simulink model "validacao_dados_degrau"  (R2021a)
settings: Solver=ode45  StartTime=0.0  StopTime=0.7  RelTol=1e-3
values from neighbouring files (symbols this model uses):
  tau_area = A0 / y_inf    [labeca_02_validacao_26_09.m]
  tau_nep = 1/a    [labeca_02_validacao_26_09.m]
undefined symbols (not defined in the file or in its folder): K_degrau
settings Model: Creator=Guilherme  LastModifiedBy=Guilherme
settings DebuggingCC: UnconnectedInputMsg=none  UnconnectedOutputMsg=none  UnconnectedLineMsg=none
settings ModelReferenceCC: EnableRefExpFcnMdlSchedulingChecks=off
settings RTWCC: Description=Generic Real-Time Target  GPUComputeCapability=5.0  DLArmComputeVersion=20.02.1

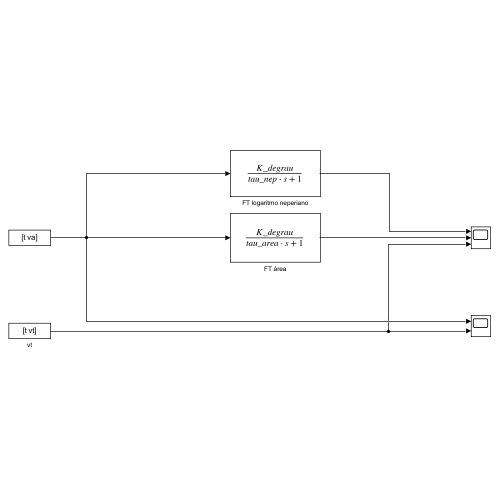
[thumbnail: Simulink's stored preview of the top-level diagram]
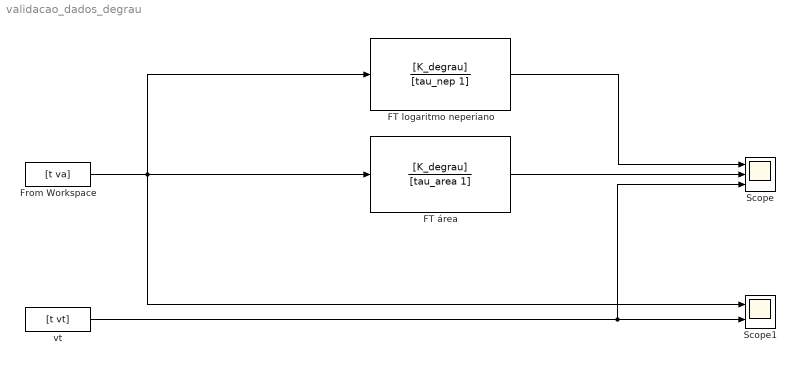
== system validacao_dados_degrau ==
  FT logaritmo neperiano : TransferFcn  Numerator=[K_degrau]  Denominator=[tau_nep 1]
  FT área : TransferFcn  Numerator=[K_degrau]  Denominator=[tau_area 1]
  From Workspace : FromWorkspace  VariableName=[t va]
  Scope : Scope  NumInputPorts=3
  Scope1 : Scope  NumInputPorts=2
  vt : FromWorkspace  VariableName=[t vt]
  wires:
  From Workspace/1 -> Scope1/1, FT área/1, FT logaritmo neperiano/1
  vt/1 -> Scope/3, Scope1/2
  FT área/1 -> Scope/2
  FT logaritmo neperiano/1 -> Scope/1
